simulink library "sm_rollerV_lib_underc_elem"  (R2026a)
settings: Solver=VariableStepAuto
undefined symbols (not defined in the file): Excv, idler_rolling_rad, roller_lower_rolling_rad, S1, S2, sprk_rolling_rad, X, Y, Z
libraries: sm_lib x42, $bdroot x10
(part 1 of 2)
Description:
  | Copyright 2024-2026 The MathWorks, Inc.
settings Model: Creator=smiller  LastModifiedBy=smiller

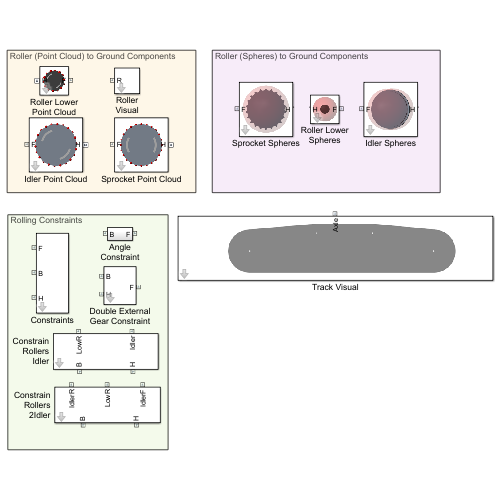
[thumbnail: Simulink's stored preview of the top-level diagram]
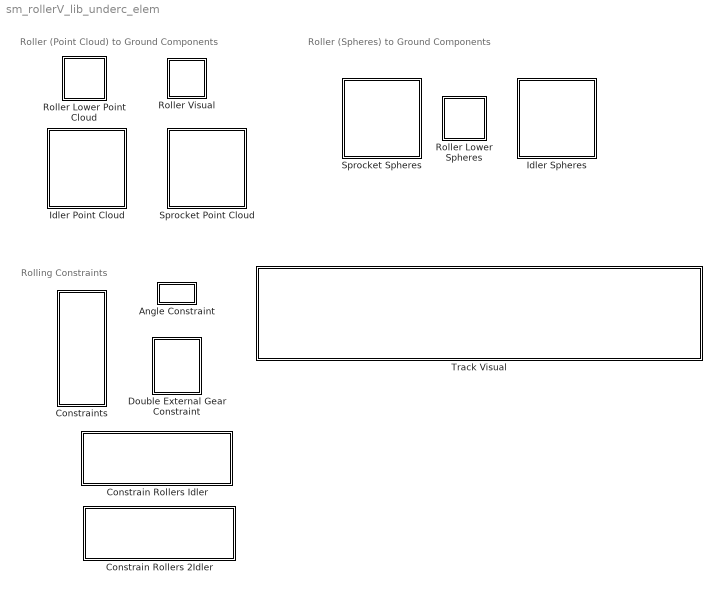
== system sm_rollerV_lib_underc_elem ==
  note: Roller (Point Cloud) to Ground Components
  note: Roller (Spheres) to Ground Components
  note: Rolling Constraints
  Angle Constraint : Subsystem
  Constrain Rollers 2Idler : Subsystem  mask(Constrain Sprocket, Lower Rollers, and Idler){sprk_rolling_rad=sprk_rolling_rad, roller_lower_rolling_rad=roller_lower_rolling_rad, idlerF_rolling_rad=idler_rolling_rad, idlerR_rolling_rad=idler_rolling_rad}
      mask prompts: sprk_rolling_rad "Sprocket Rolling Radius (m)"; roller_lower_rolling_rad "Lower Roller Rolling Radius (m)"; idlerF_rolling_rad "Front Idler Rolling Radius (m)"; idlerR_rolling_rad "Rear Idler Rolling Radius (m)"
      mask help: Model connects all required constraints to ensure sprocket, lower rollers, and idlers will spin at speeds consistent with the condition that they are all connected by the track. This enables abstract modeling of a track drive when the track drive is not present by constraining the rotation of all rolling elements that touch the ground
  Constrain Rollers Idler : Subsystem  mask(Constrain Sprocket, Lower Rollers, and Idler){sprk_rolling_rad=sprk_rolling_rad, roller_lower_rolling_rad=roller_lower_rolling_rad, idler_rolling_rad=idler_rolling_rad}
      mask prompts: sprk_rolling_rad "Sprocket Rolling Radius (m)"; roller_lower_rolling_rad "Lower Roller Rolling Radius (m)"; idler_rolling_rad "Idler Rolling Radius (m)"
      mask help: Model connects all required constraints to ensure sprocket, lower rollers, and idlers will spin at speeds consistent with the condition that they are all connected by the track. This enables abstract modeling of a track drive when the track drive is not present by constraining the rotation of all rolling elements that touch the ground
  Constraints : Subsystem  mask(Common Gear Assembly Constraints){popup_gear_type=Internal, b_gear_pd=0.3*2, f_gear_pd=0.1*2, b_visc_frict=0, f_visc_frict=0}
      mask prompts: popup_gear_type "Gear Type"
      mask help: Model connects all required constraints for a common gear assembly. Contains two Revolute Joints and a Common Gear Constraint, all oriented and positioned according to the Common Gear Constraint requirements.
      mask init:
      | gear_constr_type = get_param(gcb,'popup_gear_type');
      | set_param([gcb '/Common Gear Constraint'],'GearType',gear_constr_type);
      | if(strcmpi(gear_constr_type,'External'))
      |     gear_axis_offset = (f_gear_pd+b_gear_pd)/2;
      | else
      |     gear_axis_offset = (f_gear_pd-b_gear_pd)/2;
      | end
      mask TypeOptions popup_gear_type: External | Internal
      mask DialogControl Control3 Prompt: Gear B
      mask DialogControl Control4 Prompt: Gear F
      mask DialogControl Control5 Prompt: Pitch Diameter (m)
      mask DialogControl Control6 Prompt: Bearing Friction N*m/(deg/s)
  Double External Gear Constraint : Subsystem  mask(Constrain Sprocket, Lower Rollers, and Idler){gear_b_rad=0.3, gear_f_rad=0.1, gear_b_d=0, gear_f_d=0}
      mask prompts: gear_b_rad "Pitch Radius Gear B (m)"; gear_f_rad "Pitch Radius Gear F (m)"; gear_b_d "Bearing Friction B N*m/(deg/s)"; gear_f_d "Bearing Friction F N*m/(deg/s)"
      mask help: Model connects all required constraints to ensure base and follower spin in the same direction at a ratio consistent with their radii. This is an alternate to the Internal Common Gear Constraint.
  Idler Point Cloud : Subsystem  mask(Idler){idler_rad=Excv.Idler.rad, idler_len=Excv.Idler.len, idler_rho=Excv.Idler.rho, idler_clr=Excv.Idler.clr, idler_opc=Excv.Idler.opc, idler_contact_geo_ptcld=Excv.Idler.ground_contact.ptcld.pts, idler_contact_geo_rad=Excv.Idler.ground_contact.ptcld.rad, idler_contact_geo_clr=Excv.Idler.ground_contact.ptcld.clr, idler_contact_geo_opc=Excv.Idler.ground_contact.ptcld.opc, cyl_rad=Excv.Idler.ground_contact.rolling_radius, cyl_len=Excv.Shoe.w, cyl_clr=Excv.Idler.clr, cyl_opc=1, accMn=0.65, accMx=0.75, acc_clr=[0.8 0.8 0.8], acc_opc=1, lext=1e-3}
      mask prompts: idler_rad "Radius (m)"; idler_len "Length(m)"; idler_rho "Density (kg/m^3)"; idler_clr "Color [R G B] (0-1)"; idler_opc "Opacity (0-1)"; idler_contact_geo_ptcld "Point Cloud Data [x y z] (m)"; idler_contact_geo_rad "Radius (m)"; idler_contact_geo_clr "Color [R G B] (0-1)"; idler_contact_geo_opc "Opacity (0-1)"; cyl_rad "Cylinder Radius (m)"; cyl_len "Cylinder Length (m)"; cyl_clr "Cylinder Color [R G B] (0-1)"; cyl_opc "Cylinder Opacity (0-1)"; accMn "Accent Min Radius (0-1)"; accMx "Accent Max Radius (0-1)"; acc_clr "Accent Color [R G B] (0-1)"; acc_opc "Accent Opacity (0-1)"; lext "Length Extensions (m)"
      mask help: Models idler wheel used to tension the track in the undercarriage. A point ploud models contact with the ground as if the track were in place. This permits much faster simulation than modeling individual track segments.
      mask TypeOptions cyl_rad:
      | Roller
      | Visual/cyl_rad
      mask TypeOptions cyl_len:
      | Roller
      | Visual/cyl_len
      mask TypeOptions cyl_clr:
      | Roller
      | Visual/cyl_clr
      mask TypeOptions cyl_opc:
      | Roller
      | Visual/cyl_opc
      mask TypeOptions accMn:
      | Roller
      | Visual/accMn
      mask TypeOptions accMx:
      | Roller
      | Visual/accMx
      mask TypeOptions acc_clr:
      | Roller
      | Visual/acc_clr
      mask TypeOptions acc_opc:
      | Roller
      | Visual/acc_opc
      mask TypeOptions lext:
      | Roller
      | Visual/lext
      mask DialogControl cont_idler Prompt: Idler
      mask DialogControl cont_idler_contact_geo Prompt: Contact Geometry
      mask DialogControl cont_roller_vis Prompt: Roller Visual
      mask Display: image('sm_chain_idlerptcld_IMAGE.png');
  Idler Spheres : Subsystem  mask(Idler){idler_rad=Excv.Idler.rad, idler_len=Excv.Idler.len, idler_rho=Excv.Idler.rho, idler_clr=Excv.Idler.clr, idler_opc=Excv.Idler.opc, idler_rolling_rad=Excv.Idler.ground_contact.rolling_radius, idler_contact_geo_width=Excv.Shoe.w, idler_contact_geo_clr=Excv.Idler.ground_contact.sphere.clr, idler_contact_geo_opc=Excv.Idler.ground_contact.sphere.opc}
      mask prompts: idler_rad "Radius (m)"; idler_len "Length(m)"; idler_rho "Density (kg/m^3)"; idler_clr "Color [R G B] (0-1)"; idler_opc "Opacity (0-1)"; idler_rolling_rad "Idler to Ground Radius (m)"; idler_contact_geo_width "Shoe Width (m)"; idler_contact_geo_clr "Color [R G B] (0-1)"; idler_contact_geo_opc "Opacity (0-1)"
      mask help: Models idler wheel used to tension the track in the undercarriage. Spheres are used to model contact with the ground as if the track were in place. This abstract method of modeling ground contact permits significantly faster simulation.
      mask DialogControl idler_cont Prompt: Idler
      mask DialogControl cont_contact_geo_idler Prompt: Contact Geometry
      mask Display: image('sm_chain_idlersphere_IMAGE.png');
  Roller Visual : Subsystem  mask(Roller Visual Element){cyl_rad=Excv.Roller.Lower.ground_contact.rolling_radius, cyl_len=Excv.Shoe.w, accMx=0.75, accMn=0.65, lext=1e-3, cyl_clr=Excv.Roller.Lower.clr, acc_clr=[0.8 0.8 0.8], cyl_opc=1, acc_opc=1}
      mask prompts: cyl_rad "Cylinder Radius (m)"; cyl_len "Cylinder Length (m)"; accMx "Accent Max Radius (0-1)"; accMn "Accent Min Radius (0-1)"; lext "Length Extensions (m)"; cyl_clr "Cylinder Color [R G B] (0-1)"; acc_clr "Accent Color [R G B] (0-1)"; cyl_opc "Cylinder Opacity (0-1)"; acc_opc "Accent Opacity (0-1)"
      mask help: Models geometry to visualize rolling elements as cylinders. No inertia is provided by this element.
  Roller Lower Point Cloud : Subsystem  mask(Lower Roller){roller_lower_rad=Excv.Roller.Lower.rad, roller_lower_len=Excv.Roller.Lower.len, roller_lower_rho=Excv.Roller.Lower.rho, roller_lower_clr=Excv.Roller.Lower.clr, roller_lower_opc=Excv.Roller.Lower.opc, roller_lower_contgeo_ptcld=Excv.Roller.Lower.ground_contact.pts, roller_lower_contgeo_rad=Excv.Roller.Lower.ground_contact.rad, roller_lower_contgeo_clr=Excv.Roller.Lower.ground_contact.clr, roller_lower_contgeo_opc=Excv.Roller.Lower.ground_contact.opc, cyl_rad=Excv.Roller.Lower.ground_contact.rolling_radius, cyl_len=Excv.Shoe.w, cyl_clr=Excv.Roller.Lower.clr, cyl_opc=1, accMn=0.65, accMx=0.75, acc_clr=[0.8 0.8 0.8], acc_opc=1, lext=1e-3}
      mask prompts: roller_lower_rad "Radius (m)"; roller_lower_len "Length (m)"; roller_lower_rho "Density (kg/m^3)"; roller_lower_clr "Color [R G B] (0-1)"; roller_lower_opc "Opacity (0-1)"; roller_lower_contgeo_ptcld "Point Cloud [x y z] (m)"; roller_lower_contgeo_rad "Radius (m)"; roller_lower_contgeo_clr "Color [R G B] (0-1)"; roller_lower_contgeo_opc "Opacity (0-1)"; cyl_rad "Cylinder Radius (m)"; cyl_len "Cylinder Length (m)"; cyl_clr "Cylinder Color [R G B] (0-1)"; cyl_opc "Cylinder Opacity (0-1)"; accMn "Accent Min Radius (0-1)"; accMx "Accent Max Radius (0-1)"; acc_clr "Accent Color [R G B] (0-1)"; acc_opc "Accent Opacity (0-1)"; lext "Length Extensions (m)"
      mask help: Models lower roller on excavator undercarriage. A point cloud permits contact forces between the roller and the ground as if the track were in place. This abstract model permits significantly faster simulation than modeling the entire track as individual segments.
      mask TypeOptions cyl_rad: Roller Visual/cyl_rad
      mask TypeOptions cyl_len: Roller Visual/cyl_len
      mask TypeOptions cyl_clr: Roller Visual/cyl_clr
      mask TypeOptions cyl_opc: Roller Visual/cyl_opc
      mask TypeOptions accMn: Roller Visual/accMn
      mask TypeOptions accMx: Roller Visual/accMx
      mask TypeOptions acc_clr: Roller Visual/acc_clr
      mask TypeOptions acc_opc: Roller Visual/acc_opc
      mask TypeOptions lext: Roller Visual/lext
      mask DialogControl roller_lower_cont Prompt: Roller
      mask DialogControl cont_contact_geo_lower Prompt: Contact Geometry
      mask DialogControl cont_roller_vis Prompt: Roller Visual
      mask Display: image('sm_chain_rollerptcld_IMAGE.png');
  Roller Lower Spheres : Subsystem  mask(Lower Roller with Ground Contact){roller_lower_rad=Excv.Roller.Lower.rad, roller_lower_len=Excv.Roller.Lower.len, roller_lower_rho=Excv.Roller.Lower.rho, roller_lower_clr=Excv.Roller.Lower.clr, roller_lower_opc=Excv.Roller.Lower.opc, roller_lower_rolling_rad=Excv.Roller.Lower.ground_contact.rolling_radius, roller_lower_contgeo_width=Excv.Shoe.w, roller_lower_contgeo_clr=Excv.Roller.Lower.ground_contact.sphere.clr, roller_lower_contgeo_opc=Excv.Roller.Lower.ground_contact.sphere.opc}
      mask prompts: roller_lower_rad "Radius (m)"; roller_lower_len "Length (m)"; roller_lower_rho "Density (kg/m^3)"; roller_lower_clr "Color [R G B] (0-1)"; roller_lower_opc "Opacity (0-1)"; roller_lower_rolling_rad "Roller to Ground Rad (m)"; roller_lower_contgeo_width "Shoe Width (m)"; roller_lower_contgeo_clr "Color [R G B] (0-1)"; roller_lower_contgeo_opc "Opacity (0-1)"
      mask help: Models lower roller on excavator undercarriage. Spheres are used to model contact with the ground as if the track were in place. This abstract method of modeling ground contact permits significantly faster simulation.
      mask DialogControl roller_lower_cont Prompt: Roller
      mask DialogControl cont_contact_geo_lower Prompt: Contact Geometry
      mask Display: image('sm_chain_rollersphere_IMAGE.png');
  Sprocket Point Cloud : Subsystem  mask(Sprocket){sprk_xc=Excv.Sprocket.sprocket_xc, sprk_len=Excv.Sprocket.sprk_width, sprk_rho=Excv.Sprocket.density, sprk_clr=Excv.Sprocket.sprocket_clr, sprk_opc=Excv.Sprocket.sprocket_opc, sprk_contact_geo_ptcld=Excv.Sprocket.teeth_contact.ptcld.pts, sprk_contact_geo_rad=Excv.Sprocket.teeth_contact.ptcld.rad, sprk_contact_geo_clr=Excv.Sprocket.teeth_contact.ptcld.clr, sprk_contact_geo_opc=Excv.Sprocket.teeth_contact.ptcld.opc, cyl_rad=Excv.Sprocket.ground_contact.rolling_radius, cyl_len=Excv.Shoe.w, cyl_clr=Excv.Sprocket.clr, cyl_opc=1, accMn=0.65, accMx=0.75, acc_clr=[0.8 0.8 0.8], acc_opc=1, lext=1e-3}
      mask prompts: sprk_xc "Extrusion Data [x y] (m)"; sprk_len "Length (m)"; sprk_rho "Density (kg/m^3)"; sprk_clr "Color [R G B] (0-1)"; sprk_opc "Opacity (0-1)"; sprk_contact_geo_ptcld "Point Cloud Data [x y z] (m)"; sprk_contact_geo_rad "Radius (m)"; sprk_contact_geo_clr "Color [R G B] (0-1)"; sprk_contact_geo_opc "Opacity (0-1)"; cyl_rad "Cylinder Radius (m)"; cyl_len "Cylinder Length (m)"; cyl_clr "Cylinder Color [R G B] (0-1)"; cyl_opc "Cylinder Opacity (0-1)"; accMn "Accent Min Radius (0-1)"; accMx "Accent Max Radius (0-1)"; acc_clr "Accent Color [R G B] (0-1)"; acc_opc "Accent Opacity (0-1)"; lext "Length Extensions (m)"
      mask help: Models a sprocket. A point cloud models contact with the ground as if the track were in place. This permits much faster simulation than modeling individual track segments.
      mask TypeOptions sprk_xc: Extruded Solid/ExtrusionCrossSection
      mask TypeOptions sprk_len: Extruded Solid/ExtrusionLength
      mask TypeOptions sprk_rho: Extruded Solid/Density
      mask TypeOptions sprk_clr: Extruded Solid/GraphicDiffuseColor
      mask TypeOptions sprk_opc: Extruded Solid/GraphicOpacity
      mask TypeOptions sprk_contact_geo_ptcld: Point Cloud/CoordinatesMatrix
      mask TypeOptions sprk_contact_geo_rad: Point Cloud/GraphicSphereRadius
      mask TypeOptions sprk_contact_geo_clr: Point Cloud/GraphicDiffuseColor
      mask TypeOptions sprk_contact_geo_opc: Point Cloud/GraphicOpacity
      mask TypeOptions cyl_rad:
      | Roller
      | Visual/cyl_rad
      mask TypeOptions cyl_len:
      | Roller
      | Visual/cyl_len
      mask TypeOptions cyl_clr:
      | Roller
      | Visual/cyl_clr
      mask TypeOptions cyl_opc:
      | Roller
      | Visual/cyl_opc
      mask TypeOptions accMn:
      | Roller
      | Visual/accMn
      mask TypeOptions accMx:
      | Roller
      | Visual/accMx
      mask TypeOptions acc_clr:
      | Roller
      | Visual/acc_clr
      mask TypeOptions acc_opc:
      | Roller
      | Visual/acc_opc
      mask TypeOptions lext:
      | Roller
      | Visual/lext
      mask DialogControl cont_solida Prompt: Solid
      mask DialogControl cont_contact_geo Prompt: Contact Geometry
      mask DialogControl cont_roller_vis Prompt: Roller Visual
      mask Display: image('sm_chain_sprocketptcld_IMAGE.png');
  Sprocket Spheres : Subsystem  mask(Sprocket with Ground Contact (Spheres)){sprk_xc=Excv.Sprocket.sprocket_xc, sprk_len=Excv.Sprocket.sprk_width, sprk_rho=Excv.Sprocket.density, sprk_clr=Excv.Sprocket.sprocket_clr, sprk_opc=Excv.Sprocket.sprocket_opc, sprk_rolling_rad=Excv.Sprocket.ground_contact.rolling_radius, sprk_contact_geo_w=Excv.Shoe.w, sprk_contact_geo_clr=Excv.Sprocket.ground_contact.sphere.clr, sprk_contact_geo_opc=Excv.Sprocket.ground_contact.sphere.opc}
      mask prompts: sprk_xc "Extrusion Data [x y] (m)"; sprk_len "Length (m)"; sprk_rho "Density (kg/m^3)"; sprk_clr "Color [R G B] (0-1)"; sprk_opc "Opacity (0-1)"; sprk_rolling_rad "Sprocket to Ground Radius (m)"; sprk_contact_geo_w "Shoe Width (m)"; sprk_contact_geo_clr "Color [R G B] (0-1)"; sprk_contact_geo_opc "Opacity (0-1)"
      mask help: Models a sprocket. A point ploud models contact with the ground as if the track were in place. This abstract method of modeling ground contact permits much faster simulation than modeling individual track segments.Contact between the sprocket and a chain is not modeled.
      mask TypeOptions sprk_xc: Extruded Solid/ExtrusionCrossSection
      mask TypeOptions sprk_len: Extruded Solid/ExtrusionLength
      mask TypeOptions sprk_rho: Extruded Solid/Density
      mask TypeOptions sprk_clr: Extruded Solid/GraphicDiffuseColor
      mask TypeOptions sprk_opc: Extruded Solid/GraphicOpacity
      mask DialogControl cont_solid Prompt: Solid
      mask DialogControl cont_contact_geo Prompt: Contact Geometry
      mask Display: image('sm_chain_sprocketsphere_IMAGE.png');
  Track Visual : Subsystem  mask(Track Mass and Visual Element){track_m=Excv.Vis.Track.m, track_cg_offset=Excv.Vis.Track.cg, track_axle_offset_x=Excv.Frame.AxleX, track_axle_offset_y=Excv.Frame.AxleY, track_moi=Excv.Vis.Track.moi, track_poi=Excv.Vis.Track.poi, track_xc=Excv.Vis.Track.track_xc, track_w=Excv.Shoe.w, track_clr=Excv.Vis.Track.clr, track_opc=Excv.Vis.Track.opc}
      mask prompts: track_m "Mass"; track_cg_offset "CG Offset from Sprocket Ctr [x y z] (m)"; track_axle_offset_x "Axle Offset from Sprocket Ctr [x] (m)"; track_axle_offset_y "Axle Offset from Sprocket Ctr [y] (m)"; track_moi "Moments of Inertia  (kg*m^2)"; track_poi "Products of Inertia  (kg*m^2)"; track_xc "Extrusion Profile [x y] (m)"; track_w "Extrusion Length [(m)"; track_clr "Color [R G B] (0-1)"; track_opc "Opacity (0-1)"
      mask help: Models track drive as a single inertia element with an extruded solid. Displays the track in animations without modeling each segment.
      mask Display: image('sm_excv_track_visual_sideview_IMAGE.png');

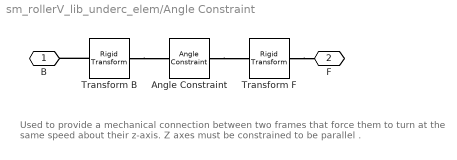
== system sm_rollerV_lib_underc_elem/Angle Constraint ==
  note: Used to provide a mechanical connection between two frames that force them to turn at the same speed about their z-axis. Z axes must be constrained to be parallel .
  Angle Constraint : sm_lib/Constraints/Angle Constraint  ConstraintType=Parallel  Angle=45  AngleUnits=deg  WrenchDir=FollowerOnBase  WrenchFrame=BaseFrame  SenseTorque=off  SenseSignedTorqueMagnitude=off
  Transform B : sm_lib/Frames and Transforms/Rigid Transform  RotationMethod=StandardAxis  FollAlignAxisA=+X  BaseAlignAxisA=+Y  FollAlignAxisB=+Y  BaseAlignAxisB=+Z  RotationStandardAxis=+X  RotationAngle=90  RotationAngleUnits=deg  RotationArbitraryAxis=[0 0 1]  RotationSequenceAxes=FollowerAxes  RotationSequence=XYX  RotationSequenceAngles=[0 0 0]  RotationSequenceAnglesUnits=deg  RotationMatrix=[1 0 0; 0 1 0; 0 0 1]  Quaternion=[1 0 0 0]  TranslationMethod=None  TranslationCartesianOffset=[0 0 0]  TranslationCartesianOffsetUnits=m  TranslationStandardAxis=+Z  TranslationStandardOffset=0  TranslationStandardOffsetUnits=m  TranslationROffset=0  TranslationROffsetUnits=m  TranslationThetaOffset=0  TranslationThetaOffsetUnits=deg  TranslationZOffset=0  TranslationZOffsetUnits=m
  Transform F : sm_lib/Frames and Transforms/Rigid Transform  RotationMethod=StandardAxis  FollAlignAxisA=+X  BaseAlignAxisA=+Y  FollAlignAxisB=+Y  BaseAlignAxisB=+Z  RotationStandardAxis=+X  RotationAngle=90  RotationAngleUnits=deg  RotationArbitraryAxis=[0 0 1]  RotationSequenceAxes=FollowerAxes  RotationSequence=XYX  RotationSequenceAngles=[0 0 0]  RotationSequenceAnglesUnits=deg  RotationMatrix=[1 0 0; 0 1 0; 0 0 1]  Quaternion=[1 0 0 0]  TranslationMethod=None  TranslationCartesianOffset=[0 0 0]  TranslationCartesianOffsetUnits=m  TranslationStandardAxis=+Z  TranslationStandardOffset=0  TranslationStandardOffsetUnits=m  TranslationROffset=0  TranslationROffsetUnits=m  TranslationThetaOffset=0  TranslationThetaOffsetUnits=deg  TranslationZOffset=0  TranslationZOffsetUnits=m
  B : PMIOPort  Side=Left
  F : PMIOPort  Port=2  Side=Right
  connections:
  Transform B/LConn1 -- B/RConn1
  Angle Constraint/RConn1 -- Transform F/RConn1
  Transform F/LConn1 -- F/RConn1
  Transform B/RConn1 -- Angle Constraint/LConn1

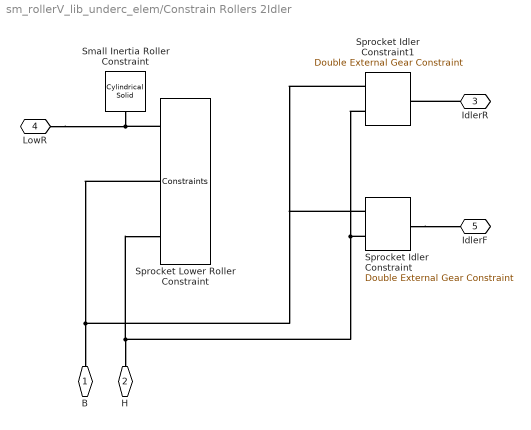
== system sm_rollerV_lib_underc_elem/Constrain Rollers 2Idler ==
  Small Inertia Roller Constraint : sm_lib/Body Elements/Cylindrical Solid  CylinderRadius=roller_lower_rolling_rad  CylinderRadiusUnits=m  CylinderLength=roller_lower_rolling_rad*0.1  CylinderLengthUnits=m  ExportEntireGeometry=off  InertiaType=CalculateFromGeometry  BasedOnType=Density  Density=1  DensityUnits=kg/m^3  Mass=1  MassUnits=kg  CenterOfMass=[0 0 0]  CenterOfMassUnits=m  MomentsOfInertia=[1 1 1]  MomentsOfInertiaUnits=kg*m^2  ProductsOfInertia=[0 0 0]  ProductsOfInertiaUnits=kg*m^2  GraphicType=FromGeometry  MarkerShape=Sphere  MarkerSize=10  GraphicVisPropType=SimpleVisualProperties  GraphicDiffuseColor=[0.5 0.5 0.5]  GraphicOpacity=0  GraphicSpecularColor=[0.5 0.5 0.5 1.0]  GraphicAmbientColor=[0.15 0.15 0.15 1.0]  GraphicEmissiveColor=[0.0 0.0 0.0 1.0]  GraphicShininess=75  DoExposeReferenceFrame=on  SerializedFrames=<Frames/>
  Sprocket Idler Constraint : $bdroot/Double External Gear Constraint  gear_b_rad=sprk_rolling_rad  gear_f_rad=idlerF_rolling_rad  gear_b_d=0  gear_f_d=0
      settings: LibrarySourceBlock=sm_excv_track_abstract_lib/Double External Constraint
  Sprocket Idler Constraint1 : $bdroot/Double External Gear Constraint  gear_b_rad=sprk_rolling_rad  gear_f_rad=idlerR_rolling_rad  gear_b_d=0  gear_f_d=0
      settings: LibrarySourceBlock=sm_excv_track_abstract_lib/Double External Constraint
  Sprocket Lower Roller Constraint : $bdroot/Constraints  popup_gear_type=Internal  b_gear_pd=sprk_rolling_rad*2  f_gear_pd=roller_lower_rolling_rad*2  b_visc_frict=0  f_visc_frict=0
  B : PMIOPort  Side=Left
  H : PMIOPort  Port=2  Side=Left
  IdlerR : PMIOPort  Port=3  Side=Right
  LowR : PMIOPort  Port=4  Side=Right
  IdlerF : PMIOPort  Port=5  Side=Right
  connections:
  Sprocket Lower Roller Constraint/LConn2 -- Sprocket Idler Constraint1/LConn1 -- Sprocket Idler Constraint/LConn1 -- B/RConn1
  Sprocket Lower Roller Constraint/LConn1 -- LowR/RConn1 -- Small Inertia Roller Constraint/RConn1
  Sprocket Idler Constraint/LConn2 -- Sprocket Lower Roller Constraint/LConn3 -- H/RConn1 -- Sprocket Idler Constraint1/LConn2
  Sprocket Idler Constraint/RConn1 -- IdlerF/RConn1
  IdlerR/RConn1 -- Sprocket Idler Constraint1/RConn1

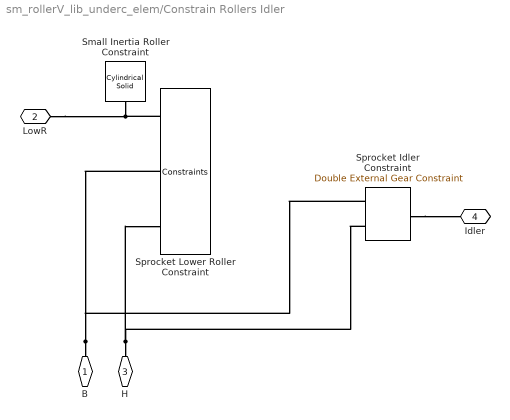
== system sm_rollerV_lib_underc_elem/Constrain Rollers Idler ==
  Small Inertia Roller Constraint : sm_lib/Body Elements/Cylindrical Solid  CylinderRadius=roller_lower_rolling_rad  CylinderRadiusUnits=m  CylinderLength=roller_lower_rolling_rad*0.1  CylinderLengthUnits=m  ExportEntireGeometry=off  InertiaType=CalculateFromGeometry  BasedOnType=Density  Density=1  DensityUnits=kg/m^3  Mass=1  MassUnits=kg  CenterOfMass=[0 0 0]  CenterOfMassUnits=m  MomentsOfInertia=[1 1 1]  MomentsOfInertiaUnits=kg*m^2  ProductsOfInertia=[0 0 0]  ProductsOfInertiaUnits=kg*m^2  GraphicType=FromGeometry  MarkerShape=Sphere  MarkerSize=10  GraphicVisPropType=SimpleVisualProperties  GraphicDiffuseColor=[0.5 0.5 0.5]  GraphicOpacity=0  GraphicSpecularColor=[0.5 0.5 0.5 1.0]  GraphicAmbientColor=[0.15 0.15 0.15 1.0]  GraphicEmissiveColor=[0.0 0.0 0.0 1.0]  GraphicShininess=75  DoExposeReferenceFrame=on  SerializedFrames=<Frames/>
  Sprocket Idler Constraint : $bdroot/Double External Gear Constraint  gear_b_rad=sprk_rolling_rad  gear_f_rad=idler_rolling_rad  gear_b_d=0  gear_f_d=0
      settings: LibrarySourceBlock=sm_excv_track_abstract_lib/Double External Constraint
  Sprocket Lower Roller Constraint : $bdroot/Constraints  popup_gear_type=Internal  b_gear_pd=sprk_rolling_rad*2  f_gear_pd=roller_lower_rolling_rad*2  b_visc_frict=0  f_visc_frict=0
  B : PMIOPort  Side=Left
  LowR : PMIOPort  Port=2  Side=Right
  H : PMIOPort  Port=3  Side=Left
  Idler : PMIOPort  Port=4  Side=Right
  connections:
  Sprocket Idler Constraint/RConn1 -- Idler/RConn1
  H/RConn1 -- Sprocket Lower Roller Constraint/LConn3 -- Sprocket Idler Constraint/LConn2
  Small Inertia Roller Constraint/RConn1 -- LowR/RConn1 -- Sprocket Lower Roller Constraint/LConn1
  B/RConn1 -- Sprocket Idler Constraint/LConn1 -- Sprocket Lower Roller Constraint/LConn2

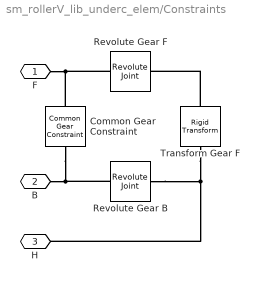
== system sm_rollerV_lib_underc_elem/Constraints ==
  Common Gear Constraint : sm_lib/Gears and Couplings/Gears/Common Gear Constraint  GearType=Internal  SpecificationType=PitchCircleRadii  CenterDistance=30  CenterDistanceUnits=cm  GearRatio=0.5  BaseGearRadius=b_gear_pd/2  BaseGearRadiusUnits=m  FollGearRadius=f_gear_pd/2  FollGearRadiusUnits=m  SensingForceTorqueDirection=FollowerOnBase  SensingForceTorqueResolutionFrame=BaseFrame  SenseForce=off  SenseTorque=off
  Revolute Gear B : sm_lib/Joints/Revolute Joint  JointMode=Normal  CompositeWrenchDir=FollowerOnBase  CompositeWrenchFrame=BaseFrame  SenseConstraintForce=off  SenseConstraintTorque=off  SenseTotalForce=off  SenseTotalTorque=off  PositionTargetSpecify=off  PositionTargetPriority=High  PositionTargetValue=0  PositionTargetValueUnits=deg  VelocityTargetSpecify=off  VelocityTargetPriority=High  VelocityTargetValue=0  VelocityTargetValueUnits=deg/s  EquilibriumPosition=0  EquilibriumPositionUnits=deg  SpringStiffness=0  SpringStiffnessUnits=N*m/deg  DampingCoefficient=b_visc_frict  DampingCoefficientUnits=N*m/(deg/s)  LowerLimitSpecify=off  LowerLimitBound=-90  LowerLimitBoundUnits=deg  LowerLimitStiffness=1e4  LowerLimitStiffnessUnits=N*m/deg  LowerLimitDamping=10  LowerLimitDampingUnits=N*m/(deg/s)  LowerLimitTransitionRegionWidth=0.1  LowerLimitTransitionRegionWidthUnits=deg  UpperLimitSpecify=off  UpperLimitBound=90  UpperLimitBoundUnits=deg  UpperLimitStiffness=1e4  UpperLimitStiffnessUnits=N*m/deg  UpperLimitDamping=10  UpperLimitDampingUnits=N*m/(deg/s)  UpperLimitTransitionRegionWidth=0.1  UpperLimitTransitionRegionWidthUnits=deg  TorqueActuationMode=NoTorque  MotionActuationMode=ComputedMotion  SensePosition=off  SenseVelocity=off  SenseAcceleration=off  SenseTorqueForce=off  SenseLowerLimitTorqueForce=off  SenseUpperLimitTorqueForce=off
  Revolute Gear F : sm_lib/Joints/Revolute Joint  JointMode=Normal  CompositeWrenchDir=FollowerOnBase  CompositeWrenchFrame=BaseFrame  SenseConstraintForce=off  SenseConstraintTorque=off  SenseTotalForce=off  SenseTotalTorque=off  PositionTargetSpecify=on  PositionTargetPriority=High  PositionTargetValue=45  PositionTargetValueUnits=deg  VelocityTargetSpecify=off  VelocityTargetPriority=High  VelocityTargetValue=0  VelocityTargetValueUnits=deg/s  EquilibriumPosition=0  EquilibriumPositionUnits=deg  SpringStiffness=0  SpringStiffnessUnits=N*m/deg  DampingCoefficient=f_visc_frict  DampingCoefficientUnits=N*m/(deg/s)  LowerLimitSpecify=off  LowerLimitBound=-90  LowerLimitBoundUnits=deg  LowerLimitStiffness=1e4  LowerLimitStiffnessUnits=N*m/deg  LowerLimitDamping=10  LowerLimitDampingUnits=N*m/(deg/s)  LowerLimitTransitionRegionWidth=0.1  LowerLimitTransitionRegionWidthUnits=deg  UpperLimitSpecify=off  UpperLimitBound=90  UpperLimitBoundUnits=deg  UpperLimitStiffness=1e4  UpperLimitStiffnessUnits=N*m/deg  UpperLimitDamping=10  UpperLimitDampingUnits=N*m/(deg/s)  UpperLimitTransitionRegionWidth=0.1  UpperLimitTransitionRegionWidthUnits=deg  TorqueActuationMode=NoTorque  MotionActuationMode=ComputedMotion  SensePosition=off  SenseVelocity=off  SenseAcceleration=off  SenseTorqueForce=off  SenseLowerLimitTorqueForce=off  SenseUpperLimitTorqueForce=off
  Transform Gear F : sm_lib/Frames and Transforms/Rigid Transform  RotationMethod=None  FollAlignAxisA=+X  BaseAlignAxisA=+Y  FollAlignAxisB=+Y  BaseAlignAxisB=+Z  RotationStandardAxis=+Z  RotationAngle=0  RotationAngleUnits=deg  RotationArbitraryAxis=[0 0 1]  RotationSequenceAxes=FollowerAxes  RotationSequence=XYX  RotationSequenceAngles=[0 0 0]  RotationSequenceAnglesUnits=deg  RotationMatrix=[1 0 0; 0 1 0; 0 0 1]  Quaternion=[1 0 0 0]  TranslationMethod=StandardAxis  TranslationCartesianOffset=[0 0 0]  TranslationCartesianOffsetUnits=m  TranslationStandardAxis=+X  TranslationStandardOffset=gear_axis_offset  TranslationStandardOffsetUnits=m  TranslationROffset=0  TranslationROffsetUnits=m  TranslationThetaOffset=0  TranslationThetaOffsetUnits=deg  TranslationZOffset=0  TranslationZOffsetUnits=m
  F : PMIOPort  Side=Left
  B : PMIOPort  Port=2  Side=Left
  H : PMIOPort  Port=3  Side=Left
  connections:
  Revolute Gear B/LConn1 -- Transform Gear F/LConn1 -- H/RConn1
  Transform Gear F/RConn1 -- Revolute Gear F/LConn1
  F/RConn1 -- Common Gear Constraint/RConn1 -- Revolute Gear F/RConn1
  B/RConn1 -- Common Gear Constraint/LConn1 -- Revolute Gear B/RConn1

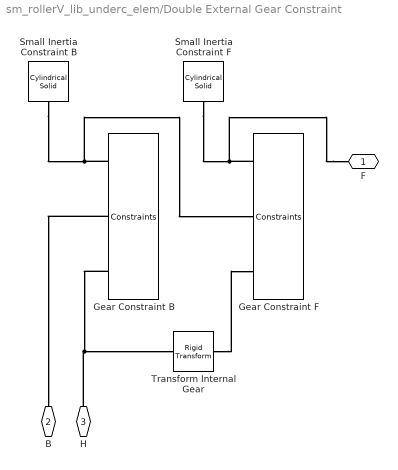
== system sm_rollerV_lib_underc_elem/Double External Gear Constraint ==
  Gear Constraint B : $bdroot/Constraints  popup_gear_type=External  b_gear_pd=gear_b_rad*2  f_gear_pd=gear_b_rad  b_visc_frict=gear_b_d  f_visc_frict=0
  Gear Constraint F : $bdroot/Constraints  popup_gear_type=External  b_gear_pd=gear_b_rad  f_gear_pd=gear_f_rad*2  b_visc_frict=0  f_visc_frict=gear_f_d
  Small Inertia Constraint B : sm_lib/Body Elements/Cylindrical Solid  CylinderRadius=gear_b_rad  CylinderRadiusUnits=m  CylinderLength=gear_b_rad*0.1  CylinderLengthUnits=m  ExportEntireGeometry=off  InertiaType=CalculateFromGeometry  BasedOnType=Density  Density=1  DensityUnits=kg/m^3  Mass=1  MassUnits=kg  CenterOfMass=[0 0 0]  CenterOfMassUnits=m  MomentsOfInertia=[1 1 1]  MomentsOfInertiaUnits=kg*m^2  ProductsOfInertia=[0 0 0]  ProductsOfInertiaUnits=kg*m^2  GraphicType=FromGeometry  MarkerShape=Sphere  MarkerSize=10  GraphicVisPropType=SimpleVisualProperties  GraphicDiffuseColor=[0.5 0.5 0.5]  GraphicOpacity=0  GraphicSpecularColor=[0.5 0.5 0.5 1.0]  GraphicAmbientColor=[0.15 0.15 0.15 1.0]  GraphicEmissiveColor=[0.0 0.0 0.0 1.0]  GraphicShininess=75  DoExposeReferenceFrame=on  SerializedFrames=<Frames/>
  Small Inertia Constraint F : sm_lib/Body Elements/Cylindrical Solid  CylinderRadius=gear_f_rad  CylinderRadiusUnits=m  CylinderLength=gear_f_rad*0.1  CylinderLengthUnits=m  ExportEntireGeometry=off  InertiaType=CalculateFromGeometry  BasedOnType=Density  Density=1  DensityUnits=kg/m^3  Mass=1  MassUnits=kg  CenterOfMass=[0 0 0]  CenterOfMassUnits=m  MomentsOfInertia=[1 1 1]  MomentsOfInertiaUnits=kg*m^2  ProductsOfInertia=[0 0 0]  ProductsOfInertiaUnits=kg*m^2  GraphicType=FromGeometry  MarkerShape=Sphere  MarkerSize=10  GraphicVisPropType=SimpleVisualProperties  GraphicDiffuseColor=[0.5 0.5 0.5]  GraphicOpacity=0  GraphicSpecularColor=[0.5 0.5 0.5 1.0]  GraphicAmbientColor=[0.15 0.15 0.15 1.0]  GraphicEmissiveColor=[0.0 0.0 0.0 1.0]  GraphicShininess=75  DoExposeReferenceFrame=on  SerializedFrames=<Frames/>
  Transform Internal Gear : sm_lib/Frames and Transforms/Rigid Transform  RotationMethod=None  FollAlignAxisA=+X  BaseAlignAxisA=+Y  FollAlignAxisB=+Y  BaseAlignAxisB=+Z  RotationStandardAxis=+Z  RotationAngle=0.0  RotationAngleUnits=deg  RotationArbitraryAxis=[0 0 1]  RotationSequenceAxes=FollowerAxes  RotationSequence=XYX  RotationSequenceAngles=[0 0 0]  RotationSequenceAnglesUnits=deg  RotationMatrix=[1 0 0; 0 1 0; 0 0 1]  Quaternion=[1 0 0 0]  TranslationMethod=StandardAxis  TranslationCartesianOffset=[0 0 0]  TranslationCartesianOffsetUnits=m  TranslationStandardAxis=+X  TranslationStandardOffset=gear_b_rad*1.5  TranslationStandardOffsetUnits=m  TranslationROffset=0  TranslationROffsetUnits=m  TranslationThetaOffset=0  TranslationThetaOffsetUnits=deg  TranslationZOffset=0  TranslationZOffsetUnits=m
  F : PMIOPort  Side=Right
  B : PMIOPort  Port=2  Side=Left
  H : PMIOPort  Port=3  Side=Left
  connections:
  Gear Constraint B/LConn2 -- B/RConn1
  Transform Internal Gear/RConn1 -- Gear Constraint F/LConn3
  Small Inertia Constraint B/RConn1 -- Gear Constraint F/LConn2 -- Gear Constraint B/LConn1
  F/RConn1 -- Small Inertia Constraint F/RConn1 -- Gear Constraint F/LConn1
  H/RConn1 -- Transform Internal Gear/LConn1 -- Gear Constraint B/LConn3

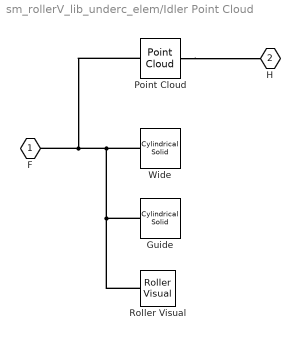
== system sm_rollerV_lib_underc_elem/Idler Point Cloud ==
  Guide : sm_lib/Body Elements/Cylindrical Solid  CylinderRadius=idler_rad*1.1  CylinderRadiusUnits=m  CylinderLength=idler_len*0.4  CylinderLengthUnits=m  ExportEntireGeometry=off  InertiaType=CalculateFromGeometry  BasedOnType=Density  Density=0  DensityUnits=kg/m^3  Mass=1  MassUnits=kg  CenterOfMass=[0 0 0]  CenterOfMassUnits=m  MomentsOfInertia=[1 1 1]  MomentsOfInertiaUnits=kg*m^2  ProductsOfInertia=[0 0 0]  ProductsOfInertiaUnits=kg*m^2  GraphicType=FromGeometry  MarkerShape=Sphere  MarkerSize=10  GraphicVisPropType=SimpleVisualProperties  GraphicDiffuseColor=idler_clr  GraphicOpacity=idler_opc  GraphicSpecularColor=[0.5 0.5 0.5 1.0]  GraphicAmbientColor=[0.15 0.15 0.15 1.0]  GraphicEmissiveColor=[0.0 0.0 0.0 1.0]  GraphicShininess=75  DoExposeReferenceFrame=on  SerializedFrames=<Frames/>
  Point Cloud : sm_lib/Curves and Surfaces/Point Cloud  CoordinatesMatrix=idler_contact_geo_ptcld  CoordinatesMatrixUnits=m  GraphicType=MarkerCloud  GraphicSphereRadius=idler_contact_geo_rad  GraphicSphereRadiusUnits=m  GraphicVisPropType=SimpleVisualProperties  GraphicDiffuseColor=idler_contact_geo_clr  GraphicOpacity=idler_contact_geo_opc  GraphicSpecularColor=[0.5 0.5 0.5 1.0]  GraphicAmbientColor=[0.15 0.15 0.15 1.0]  GraphicEmissiveColor=[0.0 0.0 0.0 1.0]  GraphicShininess=75
  Roller Visual : $bdroot/Roller Visual  cyl_rad=cyl_rad  cyl_len=cyl_len  accMx=accMx  accMn=accMn  lext=lext  cyl_clr=cyl_clr  acc_clr=acc_clr  cyl_opc=cyl_opc  acc_opc=acc_opc
  Wide : sm_lib/Body Elements/Cylindrical Solid  CylinderRadius=idler_rad  CylinderRadiusUnits=m  CylinderLength=idler_len  CylinderLengthUnits=m  ExportEntireGeometry=off  InertiaType=CalculateFromGeometry  BasedOnType=Density  Density=idler_rho  DensityUnits=kg/m^3  Mass=1  MassUnits=kg  CenterOfMass=[0 0 0]  CenterOfMassUnits=m  MomentsOfInertia=[1 1 1]  MomentsOfInertiaUnits=kg*m^2  ProductsOfInertia=[0 0 0]  ProductsOfInertiaUnits=kg*m^2  GraphicType=FromGeometry  MarkerShape=Sphere  MarkerSize=10  GraphicVisPropType=SimpleVisualProperties  GraphicDiffuseColor=idler_clr  GraphicOpacity=idler_opc  GraphicSpecularColor=[0.5 0.5 0.5 1.0]  GraphicAmbientColor=[0.15 0.15 0.15 1.0]  GraphicEmissiveColor=[0.0 0.0 0.0 1.0]  GraphicShininess=75  DoExposeReferenceFrame=on  SerializedFrames=<Frames/>
  F : PMIOPort  Side=Left
  H : PMIOPort  Port=2  Side=Right
  connections:
  F/RConn1 -- Point Cloud/LConn1 -- Guide/RConn1 -- Roller Visual/LConn1 -- Wide/RConn1
  Point Cloud/RConn1 -- H/RConn1

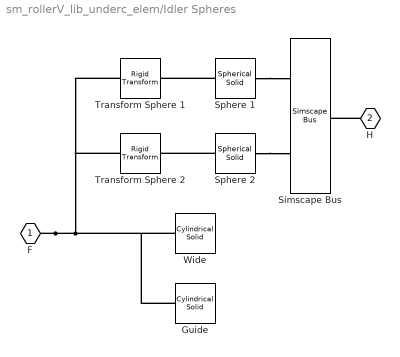
== system sm_rollerV_lib_underc_elem/Idler Spheres ==
  Guide : sm_lib/Body Elements/Cylindrical Solid  CylinderRadius=idler_rad*1.1  CylinderRadiusUnits=m  CylinderLength=idler_len*0.4  CylinderLengthUnits=m  ExportEntireGeometry=off  InertiaType=CalculateFromGeometry  BasedOnType=Density  Density=0  DensityUnits=kg/m^3  Mass=1  MassUnits=kg  CenterOfMass=[0 0 0]  CenterOfMassUnits=m  MomentsOfInertia=[1 1 1]  MomentsOfInertiaUnits=kg*m^2  ProductsOfInertia=[0 0 0]  ProductsOfInertiaUnits=kg*m^2  GraphicType=FromGeometry  MarkerShape=Sphere  MarkerSize=10  GraphicVisPropType=SimpleVisualProperties  GraphicDiffuseColor=idler_clr  GraphicOpacity=idler_opc  GraphicSpecularColor=[0.5 0.5 0.5 1.0]  GraphicAmbientColor=[0.15 0.15 0.15 1.0]  GraphicEmissiveColor=[0.0 0.0 0.0 1.0]  GraphicShininess=75  DoExposeReferenceFrame=on  SerializedFrames=<Frames/>
  Simscape Bus : SimscapeBus  HierarchyStrings=S1;S2
  Sphere 1 : sm_lib/Body Elements/Spherical Solid  SphereRadius=idler_rolling_rad  SphereRadiusUnits=m  ExportEntireGeometry=on  InertiaType=CalculateFromGeometry  BasedOnType=Density  Density=0  DensityUnits=kg/m^3  Mass=1  MassUnits=kg  CenterOfMass=[0 0 0]  CenterOfMassUnits=m  MomentsOfInertia=[1 1 1]  MomentsOfInertiaUnits=kg*m^2  ProductsOfInertia=[0 0 0]  ProductsOfInertiaUnits=kg*m^2  GraphicType=FromGeometry  MarkerShape=Sphere  MarkerSize=10  GraphicVisPropType=SimpleVisualProperties  GraphicDiffuseColor=idler_contact_geo_clr  GraphicOpacity=idler_contact_geo_opc  GraphicSpecularColor=[0.5 0.5 0.5 1.0]  GraphicAmbientColor=[0.15 0.15 0.15 1.0]  GraphicEmissiveColor=[0.0 0.0 0.0 1.0]  GraphicShininess=75  DoExposeReferenceFrame=on  SerializedFrames=<Frames/>
  Sphere 2 : sm_lib/Body Elements/Spherical Solid  SphereRadius=idler_rolling_rad  SphereRadiusUnits=m  ExportEntireGeometry=on  InertiaType=CalculateFromGeometry  BasedOnType=Density  Density=0  DensityUnits=kg/m^3  Mass=1  MassUnits=kg  CenterOfMass=[0 0 0]  CenterOfMassUnits=m  MomentsOfInertia=[1 1 1]  MomentsOfInertiaUnits=kg*m^2  ProductsOfInertia=[0 0 0]  ProductsOfInertiaUnits=kg*m^2  GraphicType=FromGeometry  MarkerShape=Sphere  MarkerSize=10  GraphicVisPropType=SimpleVisualProperties  GraphicDiffuseColor=idler_contact_geo_clr  GraphicOpacity=idler_contact_geo_opc  GraphicSpecularColor=[0.5 0.5 0.5 1.0]  GraphicAmbientColor=[0.15 0.15 0.15 1.0]  GraphicEmissiveColor=[0.0 0.0 0.0 1.0]  GraphicShininess=75  DoExposeReferenceFrame=on  SerializedFrames=<Frames/>
  Transform Sphere 1 : sm_lib/Frames and Transforms/Rigid Transform  RotationMethod=None  FollAlignAxisA=+X  BaseAlignAxisA=+Y  FollAlignAxisB=+Y  BaseAlignAxisB=+Z  RotationStandardAxis=+Z  RotationAngle=0.0  RotationAngleUnits=deg  RotationArbitraryAxis=[0 0 1]  RotationSequenceAxes=FollowerAxes  RotationSequence=XYX  RotationSequenceAngles=[0 0 0]  RotationSequenceAnglesUnits=deg  RotationMatrix=[1 0 0; 0 1 0; 0 0 1]  Quaternion=[1 0 0 0]  TranslationMethod=StandardAxis  TranslationCartesianOffset=[0 0 0]  TranslationCartesianOffsetUnits=m  TranslationStandardAxis=+Z  TranslationStandardOffset=idler_contact_geo_width/2  TranslationStandardOffsetUnits=m  TranslationROffset=0  TranslationROffsetUnits=m  TranslationThetaOffset=0  TranslationThetaOffsetUnits=deg  TranslationZOffset=0  TranslationZOffsetUnits=m
  Transform Sphere 2 : sm_lib/Frames and Transforms/Rigid Transform  RotationMethod=None  FollAlignAxisA=+X  BaseAlignAxisA=+Y  FollAlignAxisB=+Y  BaseAlignAxisB=+Z  RotationStandardAxis=+Z  RotationAngle=0.0  RotationAngleUnits=deg  RotationArbitraryAxis=[0 0 1]  RotationSequenceAxes=FollowerAxes  RotationSequence=XYX  RotationSequenceAngles=[0 0 0]  RotationSequenceAnglesUnits=deg  RotationMatrix=[1 0 0; 0 1 0; 0 0 1]  Quaternion=[1 0 0 0]  TranslationMethod=StandardAxis  TranslationCartesianOffset=[0 0 0]  TranslationCartesianOffsetUnits=m  TranslationStandardAxis=+Z  TranslationStandardOffset=-idler_contact_geo_width/2  TranslationStandardOffsetUnits=m  TranslationROffset=0  TranslationROffsetUnits=m  TranslationThetaOffset=0  TranslationThetaOffsetUnits=deg  TranslationZOffset=0  TranslationZOffsetUnits=m
  Wide : sm_lib/Body Elements/Cylindrical Solid  CylinderRadius=idler_rad  CylinderRadiusUnits=m  CylinderLength=idler_len  CylinderLengthUnits=m  ExportEntireGeometry=off  InertiaType=CalculateFromGeometry  BasedOnType=Density  Density=idler_rho  DensityUnits=kg/m^3  Mass=1  MassUnits=kg  CenterOfMass=[0 0 0]  CenterOfMassUnits=m  MomentsOfInertia=[1 1 1]  MomentsOfInertiaUnits=kg*m^2  ProductsOfInertia=[0 0 0]  ProductsOfInertiaUnits=kg*m^2  GraphicType=FromGeometry  MarkerShape=Sphere  MarkerSize=10  GraphicVisPropType=SimpleVisualProperties  GraphicDiffuseColor=idler_clr  GraphicOpacity=idler_opc  GraphicSpecularColor=[0.5 0.5 0.5 1.0]  GraphicAmbientColor=[0.15 0.15 0.15 1.0]  GraphicEmissiveColor=[0.0 0.0 0.0 1.0]  GraphicShininess=75  DoExposeReferenceFrame=on  SerializedFrames=<Frames/>
  F : PMIOPort  Side=Left
  H : PMIOPort  Port=2  Side=Right
  connections:
  Sphere 1/LConn1 -- Simscape Bus/LConn1
  Sphere 2/LConn1 -- Simscape Bus/LConn2
  Sphere 1/RConn1 -- Transform Sphere 1/RConn1
  H/RConn1 -- Simscape Bus/RConn1
  Sphere 2/RConn1 -- Transform Sphere 2/RConn1
  F/RConn1 -- Wide/RConn1 -- Guide/RConn1 -- Transform Sphere 2/LConn1 -- Transform Sphere 1/LConn1

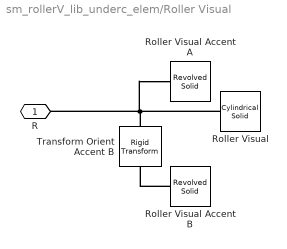
== system sm_rollerV_lib_underc_elem/Roller Visual ==
  Roller Visual : sm_lib/Body Elements/Cylindrical Solid  CylinderRadius=cyl_rad  CylinderRadiusUnits=m  CylinderLength=cyl_len+lext  CylinderLengthUnits=m  ExportEntireGeometry=off  InertiaType=CalculateFromGeometry  BasedOnType=Density  Density=0  DensityUnits=kg/m^3  Mass=1  MassUnits=kg  CenterOfMass=[0 0 0]  CenterOfMassUnits=m  MomentsOfInertia=[1 1 1]  MomentsOfInertiaUnits=kg*m^2  ProductsOfInertia=[0 0 0]  ProductsOfInertiaUnits=kg*m^2  GraphicType=FromGeometry  MarkerShape=Sphere  MarkerSize=10  GraphicVisPropType=SimpleVisualProperties  GraphicDiffuseColor=cyl_clr  GraphicOpacity=cyl_opc  GraphicSpecularColor=[0.5 0.5 0.5 1.0]  GraphicAmbientColor=[0.15 0.15 0.15 1.0]  GraphicEmissiveColor=[0.0 0.0 0.0 1.0]  GraphicShininess=75  DoExposeReferenceFrame=on  SerializedFrames=<Frames/>
  Roller Visual Accent A : sm_lib/Body Elements/Revolved Solid  RevolutionCrossSection=[accMn 0.5; accMn -0.5; accMx -0.5; accMx 0.5].*[cyl_rad cyl_len+lext*2]  RevolutionCrossSectionUnits=m  RevolutionExtent=Custom  RevolutionAngle=60  RevolutionAngleUnits=deg  ExportConvexHullGeometry=off  InertiaType=CalculateFromGeometry  BasedOnType=Density  Density=0  DensityUnits=kg/m^3  Mass=1  MassUnits=kg  CenterOfMass=[0 0 0]  CenterOfMassUnits=m  MomentsOfInertia=[1 1 1]  MomentsOfInertiaUnits=kg*m^2  ProductsOfInertia=[0 0 0]  ProductsOfInertiaUnits=kg*m^2  GraphicType=FromGeometry  MarkerShape=Sphere  MarkerSize=10  GraphicVisPropType=SimpleVisualProperties  GraphicDiffuseColor=acc_clr  GraphicOpacity=acc_opc  GraphicSpecularColor=[0.5 0.5 0.5 1.0]  GraphicAmbientColor=[0.15 0.15 0.15 1.0]  GraphicEmissiveColor=[0.0 0.0 0.0 1.0]  GraphicShininess=75  DoExposeReferenceFrame=on  SerializedFrames=<Frames/>
  Roller Visual Accent B : sm_lib/Body Elements/Revolved Solid  RevolutionCrossSection=[accMn 0.5; accMn -0.5; accMx -0.5; accMx 0.5].*[cyl_rad cyl_len+lext*2]  RevolutionCrossSectionUnits=m  RevolutionExtent=Custom  RevolutionAngle=60  RevolutionAngleUnits=deg  ExportConvexHullGeometry=off  InertiaType=CalculateFromGeometry  BasedOnType=Density  Density=0  DensityUnits=kg/m^3  Mass=1  MassUnits=kg  CenterOfMass=[0 0 0]  CenterOfMassUnits=m  MomentsOfInertia=[1 1 1]  MomentsOfInertiaUnits=kg*m^2  ProductsOfInertia=[0 0 0]  ProductsOfInertiaUnits=kg*m^2  GraphicType=FromGeometry  MarkerShape=Sphere  MarkerSize=10  GraphicVisPropType=SimpleVisualProperties  GraphicDiffuseColor=acc_clr  GraphicOpacity=acc_opc  GraphicSpecularColor=[0.5 0.5 0.5 1.0]  GraphicAmbientColor=[0.15 0.15 0.15 1.0]  GraphicEmissiveColor=[0.0 0.0 0.0 1.0]  GraphicShininess=75  DoExposeReferenceFrame=on  SerializedFrames=<Frames/>
  Transform Orient Accent B : sm_lib/Frames and Transforms/Rigid Transform  RotationMethod=StandardAxis  FollAlignAxisA=+X  BaseAlignAxisA=+Y  FollAlignAxisB=+Y  BaseAlignAxisB=+Z  RotationStandardAxis=+Z  RotationAngle=180  RotationAngleUnits=deg  RotationArbitraryAxis=[0 0 1]  RotationSequenceAxes=FollowerAxes  RotationSequence=XYX  RotationSequenceAngles=[0 0 0]  RotationSequenceAnglesUnits=deg  RotationMatrix=[1 0 0; 0 1 0; 0 0 1]  Quaternion=[1 0 0 0]  TranslationMethod=None  TranslationCartesianOffset=[0 0 0]  TranslationCartesianOffsetUnits=m  TranslationStandardAxis=+Z  TranslationStandardOffset=0  TranslationStandardOffsetUnits=m  TranslationROffset=0  TranslationROffsetUnits=m  TranslationThetaOffset=0  TranslationThetaOffsetUnits=deg  TranslationZOffset=0  TranslationZOffsetUnits=m
  R : PMIOPort  Side=Left
  connections:
  R/RConn1 -- Roller Visual Accent A/RConn1 -- Roller Visual/RConn1 -- Transform Orient Accent B/LConn1
  Roller Visual Accent B/RConn1 -- Transform Orient Accent B/RConn1

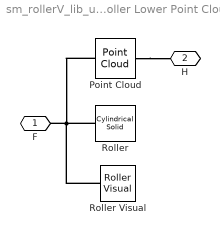
== system sm_rollerV_lib_underc_elem/Roller Lower Point Cloud ==
  Point Cloud : sm_lib/Curves and Surfaces/Point Cloud  CoordinatesMatrix=roller_lower_contgeo_ptcld  CoordinatesMatrixUnits=m  GraphicType=MarkerCloud  GraphicSphereRadius=roller_lower_contgeo_rad  GraphicSphereRadiusUnits=m  GraphicVisPropType=SimpleVisualProperties  GraphicDiffuseColor=roller_lower_contgeo_clr  GraphicOpacity=roller_lower_contgeo_opc  GraphicSpecularColor=[0.5 0.5 0.5 1.0]  GraphicAmbientColor=[0.15 0.15 0.15 1.0]  GraphicEmissiveColor=[0.0 0.0 0.0 1.0]  GraphicShininess=75
  Roller : sm_lib/Body Elements/Cylindrical Solid  CylinderRadius=roller_lower_rad  CylinderRadiusUnits=m  CylinderLength=roller_lower_len  CylinderLengthUnits=m  ExportEntireGeometry=off  InertiaType=CalculateFromGeometry  BasedOnType=Density  Density=roller_lower_rho  DensityUnits=kg/m^3  Mass=1  MassUnits=kg  CenterOfMass=[0 0 0]  CenterOfMassUnits=m  MomentsOfInertia=[1 1 1]  MomentsOfInertiaUnits=kg*m^2  ProductsOfInertia=[0 0 0]  ProductsOfInertiaUnits=kg*m^2  GraphicType=FromGeometry  MarkerShape=Sphere  MarkerSize=10  GraphicVisPropType=SimpleVisualProperties  GraphicDiffuseColor=roller_lower_clr  GraphicOpacity=roller_lower_opc  GraphicSpecularColor=[0.5 0.5 0.5 1.0]  GraphicAmbientColor=[0.15 0.15 0.15 1.0]  GraphicEmissiveColor=[0.0 0.0 0.0 1.0]  GraphicShininess=75  DoExposeReferenceFrame=on  SerializedFrames=<Frames/>
  Roller Visual : $bdroot/Roller Visual  cyl_rad=cyl_rad  cyl_len=cyl_len  accMx=accMx  accMn=accMn  lext=lext  cyl_clr=cyl_clr  acc_clr=acc_clr  cyl_opc=cyl_opc  acc_opc=acc_opc
  F : PMIOPort  Side=Left
  H : PMIOPort  Port=2  Side=Right
  connections:
  Roller/RConn1 -- Roller Visual/LConn1 -- F/RConn1 -- Point Cloud/LConn1
  Point Cloud/RConn1 -- H/RConn1

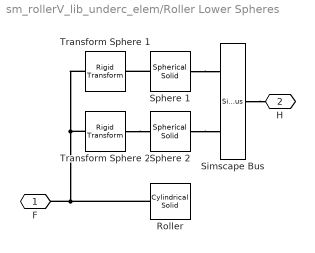
== system sm_rollerV_lib_underc_elem/Roller Lower Spheres ==
  Roller : sm_lib/Body Elements/Cylindrical Solid  CylinderRadius=roller_lower_rad  CylinderRadiusUnits=m  CylinderLength=roller_lower_len  CylinderLengthUnits=m  ExportEntireGeometry=off  InertiaType=CalculateFromGeometry  BasedOnType=Density  Density=roller_lower_rho  DensityUnits=kg/m^3  Mass=1  MassUnits=kg  CenterOfMass=[0 0 0]  CenterOfMassUnits=m  MomentsOfInertia=[1 1 1]  MomentsOfInertiaUnits=kg*m^2  ProductsOfInertia=[0 0 0]  ProductsOfInertiaUnits=kg*m^2  GraphicType=FromGeometry  MarkerShape=Sphere  MarkerSize=10  GraphicVisPropType=SimpleVisualProperties  GraphicDiffuseColor=roller_lower_clr  GraphicOpacity=roller_lower_opc  GraphicSpecularColor=[0.5 0.5 0.5 1.0]  GraphicAmbientColor=[0.15 0.15 0.15 1.0]  GraphicEmissiveColor=[0.0 0.0 0.0 1.0]  GraphicShininess=75  DoExposeReferenceFrame=on  SerializedFrames=<Frames/>
  Simscape Bus : SimscapeBus  HierarchyStrings=S1;S2
  Sphere 1 : sm_lib/Body Elements/Spherical Solid  SphereRadius=roller_lower_rolling_rad  SphereRadiusUnits=m  ExportEntireGeometry=on  InertiaType=CalculateFromGeometry  BasedOnType=Density  Density=0  DensityUnits=kg/m^3  Mass=1  MassUnits=kg  CenterOfMass=[0 0 0]  CenterOfMassUnits=m  MomentsOfInertia=[1 1 1]  MomentsOfInertiaUnits=kg*m^2  ProductsOfInertia=[0 0 0]  ProductsOfInertiaUnits=kg*m^2  GraphicType=FromGeometry  MarkerShape=Sphere  MarkerSize=10  GraphicVisPropType=SimpleVisualProperties  GraphicDiffuseColor=roller_lower_contgeo_clr  GraphicOpacity=roller_lower_contgeo_opc  GraphicSpecularColor=[0.5 0.5 0.5 1.0]  GraphicAmbientColor=[0.15 0.15 0.15 1.0]  GraphicEmissiveColor=[0.0 0.0 0.0 1.0]  GraphicShininess=75  DoExposeReferenceFrame=on  SerializedFrames=<Frames/>
  Sphere 2 : sm_lib/Body Elements/Spherical Solid  SphereRadius=roller_lower_rolling_rad  SphereRadiusUnits=m  ExportEntireGeometry=on  InertiaType=CalculateFromGeometry  BasedOnType=Density  Density=0  DensityUnits=kg/m^3  Mass=1  MassUnits=kg  CenterOfMass=[0 0 0]  CenterOfMassUnits=m  MomentsOfInertia=[1 1 1]  MomentsOfInertiaUnits=kg*m^2  ProductsOfInertia=[0 0 0]  ProductsOfInertiaUnits=kg*m^2  GraphicType=FromGeometry  MarkerShape=Sphere  MarkerSize=10  GraphicVisPropType=SimpleVisualProperties  GraphicDiffuseColor=roller_lower_contgeo_clr  GraphicOpacity=roller_lower_contgeo_opc  GraphicSpecularColor=[0.5 0.5 0.5 1.0]  GraphicAmbientColor=[0.15 0.15 0.15 1.0]  GraphicEmissiveColor=[0.0 0.0 0.0 1.0]  GraphicShininess=75  DoExposeReferenceFrame=on  SerializedFrames=<Frames/>
  Transform Sphere 1 : sm_lib/Frames and Transforms/Rigid Transform  RotationMethod=None  FollAlignAxisA=+X  BaseAlignAxisA=+Y  FollAlignAxisB=+Y  BaseAlignAxisB=+Z  RotationStandardAxis=+Z  RotationAngle=0.0  RotationAngleUnits=deg  RotationArbitraryAxis=[0 0 1]  RotationSequenceAxes=FollowerAxes  RotationSequence=XYX  RotationSequenceAngles=[0 0 0]  RotationSequenceAnglesUnits=deg  RotationMatrix=[1 0 0; 0 1 0; 0 0 1]  Quaternion=[1 0 0 0]  TranslationMethod=StandardAxis  TranslationCartesianOffset=[0 0 0]  TranslationCartesianOffsetUnits=m  TranslationStandardAxis=+Z  TranslationStandardOffset=roller_lower_contgeo_width/2  TranslationStandardOffsetUnits=m  TranslationROffset=0  TranslationROffsetUnits=m  TranslationThetaOffset=0  TranslationThetaOffsetUnits=deg  TranslationZOffset=0  TranslationZOffsetUnits=m
  Transform Sphere 2 : sm_lib/Frames and Transforms/Rigid Transform  RotationMethod=None  FollAlignAxisA=+X  BaseAlignAxisA=+Y  FollAlignAxisB=+Y  BaseAlignAxisB=+Z  RotationStandardAxis=+Z  RotationAngle=0.0  RotationAngleUnits=deg  RotationArbitraryAxis=[0 0 1]  RotationSequenceAxes=FollowerAxes  RotationSequence=XYX  RotationSequenceAngles=[0 0 0]  RotationSequenceAnglesUnits=deg  RotationMatrix=[1 0 0; 0 1 0; 0 0 1]  Quaternion=[1 0 0 0]  TranslationMethod=StandardAxis  TranslationCartesianOffset=[0 0 0]  TranslationCartesianOffsetUnits=m  TranslationStandardAxis=+Z  TranslationStandardOffset=-roller_lower_contgeo_width/2  TranslationStandardOffsetUnits=m  TranslationROffset=0  TranslationROffsetUnits=m  TranslationThetaOffset=0  TranslationThetaOffsetUnits=deg  TranslationZOffset=0  TranslationZOffsetUnits=m
  F : PMIOPort  Side=Left
  H : PMIOPort  Port=2  Side=Right
  connections:
  Transform Sphere 2/RConn1 -- Sphere 2/RConn1
  Sphere 2/LConn1 -- Simscape Bus/LConn2
  Sphere 1/LConn1 -- Simscape Bus/LConn1
  Sphere 1/RConn1 -- Transform Sphere 1/RConn1
  Simscape Bus/RConn1 -- H/RConn1
  Transform Sphere 2/LConn1 -- Transform Sphere 1/LConn1 -- F/RConn1 -- Roller/RConn1
